simulink model "motor_model"  (R2014b)
settings: Solver=ode45  StartTime=0.0  StopTime=2  RelTol=1e-3
values from neighbouring files (symbols this model uses):
  act_limit = 60    [motor_params.m]
  noise_amp = 0    [motor_params.m]
  noise_freq = 300*2*pi    (= 1884.95559215)    [motor_params.m]
undefined symbols (not defined in the file or in its folder): lead_k, lead_pole, lead_zero, P
settings Model: Creator=dhoelzle  LastModifiedBy=dhoelzle

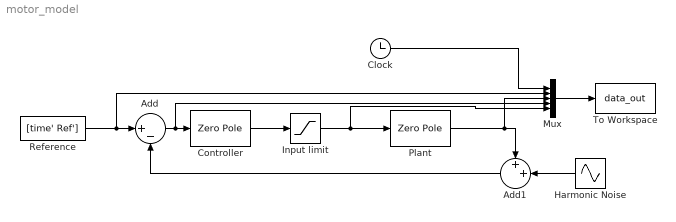
== system motor_model ==
  Add : Sum  Inputs=|+-
  Add1 : Sum  Inputs=++|
  Clock : Clock
  Controller : ZeroPole  Zeros=[lead_zero]  Poles=[lead_pole]  Gain=[lead_k]
  Harmonic Noise : Sin  Amplitude=noise_amp  Frequency=noise_freq  SampleTime=0
  Input limit : Saturate  UpperLimit=act_limit  LowerLimit=-act_limit
  Mux : Mux  Inputs=5
  Plant : ZeroPole  Zeros=cell2mat(P.z)  Poles=cell2mat(P.p)  Gain=P.k
  Reference : FromWorkspace  VariableName=[time' Ref']  SampleTime=0  OutputAfterFinalValue=Holding final value
  To Workspace : ToWorkspace  VariableName=data_out  SampleTime=-1
  wires:
  Controller/1 -> Input limit/1
  Add/1 -> Mux/4, Controller/1
  Reference/1 -> Mux/2, Add/1
  Clock/1 -> Mux/1
  Mux/1 -> To Workspace/1
  Input limit/1 -> Mux/5, Plant/1
  Add1/1 -> Add/2
  Harmonic Noise/1 -> Add1/2
  Plant/1 -> Mux/3, Add1/1
